simulink model "test_mdl_NI"  (R2018a)
settings: Solver=VariableStepAuto  StartTime=0.0  StopTime=10.0  RelTol=1e-3
(part 19 of 24)

== system test_mdl_NI/CAN_Signal/GWM/Other_GWMTx/Cluster_Info1_FD1 ==
  in : Inport
  AccDeny_B_RqIpc : Subsystem
  AccEnbl_B_RqDrv : Subsystem
  BulbChkActv_B_Stat : Subsystem
  DrvPerfMde_D_Rq : Subsystem
  DrvSlipCtlMde_B_Rq2 : Subsystem
  DrvSlipCtlMde_D_Rq : Subsystem
  EmgcyCallAsstMykey_Rq : Subsystem
  EngIdlShutDown_B_RqDrv : Subsystem
  EngOilLife_B_RqReset : Subsystem
  Fda_B_Stat : Subsystem
  FrostWarn_D_Stat : Subsystem
  HsaMde_D_Rq : Subsystem
  KeyTypeChngMykey_D_Rq : Subsystem
  LscmbbStat_B_Actl : Subsystem
  ManRgen_D_Rq : Subsystem
  MetricActvTe_B_Actl : Subsystem
  MetricActv_B_Actl : Subsystem
  NtrlTowMdeEnbl_B_RqDrv : Subsystem
  OdometerMasterValue : Subsystem
  ParkDetect_Stat : Subsystem
  Power_Liftgate_Mode_Cmd : Subsystem
  PrkLckCtlEnbl_D_RqIpc : Subsystem
  PtDrvMde_D_Rq : Subsystem
  ReducedGuard_D_Rq : Subsystem
  StopStrtDrvMde_D_RqMnu : Subsystem
  TRAILER_BRAKE_CONFIG : Subsystem
  TRLR_SWAY_CONFIG_CMD : Subsystem
  TrlrBrkMde_D_Rq : Subsystem
  bus_creator : BusCreator  Inputs=29
  bus_selector : BusSelector  OutputSignals=AccDeny_B_RqIpc,AccEnbl_B_RqDrv,BulbChkActv_B_Stat,DrvPerfMde_D_Rq,DrvSlipCtlMde_B_Rq2,DrvSlipCtlMde_D_Rq,EmgcyCallAsstMykey_Rq,EngIdlShutDown_B_RqDrv,EngOilLife_B_RqReset,Fda_B_Stat,FrostWarn_D_Stat,HsaMde_D_Rq,KeyTypeChngMykey_D_Rq,LscmbbStat_B_Actl,ManRgen_D_Rq,MetricActvTe_B_Actl,MetricActv_B_Actl,NtrlTowMdeEnbl_B_RqDrv,OdometerMasterValue,ParkDetect_Stat,Power_Liftgate_Mode_Cmd,PrkLckCtlEnbl_D_RqIpc,PtDrvMde_D_Rq,ReducedGuard_D_Rq,StopStrtDrvMde_D_RqMnu,TRAILER_BRAKE_CONFIG,TRLR_SWAY_CONFIG_CMD,TrlrBrkMde_D_Rq,ePRNDL_MODE
  ePRNDL_MODE : Subsystem
  out_port : Outport
  wires:
  bus_creator/1 -> out_port/1  "Cluster_Info1_FD1"
  AccDeny_B_RqIpc/1(out) -> bus_creator/1  "AccDeny_B_RqIpc"
  AccEnbl_B_RqDrv/1(out) -> bus_creator/2  "AccEnbl_B_RqDrv"
  BulbChkActv_B_Stat/1(out) -> bus_creator/3  "BulbChkActv_B_Stat"
  DrvPerfMde_D_Rq/1(out) -> bus_creator/4  "DrvPerfMde_D_Rq"
  DrvSlipCtlMde_B_Rq2/1(out) -> bus_creator/5  "DrvSlipCtlMde_B_Rq2"
  DrvSlipCtlMde_D_Rq/1(out) -> bus_creator/6  "DrvSlipCtlMde_D_Rq"
  EmgcyCallAsstMykey_Rq/1(out) -> bus_creator/7  "EmgcyCallAsstMykey_Rq"
  EngIdlShutDown_B_RqDrv/1(out) -> bus_creator/8  "EngIdlShutDown_B_RqDrv"
  EngOilLife_B_RqReset/1(out) -> bus_creator/9  "EngOilLife_B_RqReset"
  Fda_B_Stat/1(out) -> bus_creator/10  "Fda_B_Stat"
  FrostWarn_D_Stat/1(out) -> bus_creator/11  "FrostWarn_D_Stat"
  HsaMde_D_Rq/1(out) -> bus_creator/12  "HsaMde_D_Rq"
  KeyTypeChngMykey_D_Rq/1(out) -> bus_creator/13  "KeyTypeChngMykey_D_Rq"
  LscmbbStat_B_Actl/1(out) -> bus_creator/14  "LscmbbStat_B_Actl"
  ManRgen_D_Rq/1(out) -> bus_creator/15  "ManRgen_D_Rq"
  MetricActvTe_B_Actl/1(out) -> bus_creator/16  "MetricActvTe_B_Actl"
  MetricActv_B_Actl/1(out) -> bus_creator/17  "MetricActv_B_Actl"
  NtrlTowMdeEnbl_B_RqDrv/1(out) -> bus_creator/18  "NtrlTowMdeEnbl_B_RqDrv"
  OdometerMasterValue/1(out) -> bus_creator/19  "OdometerMasterValue"
  ParkDetect_Stat/1(out) -> bus_creator/20  "ParkDetect_Stat"
  Power_Liftgate_Mode_Cmd/1(out) -> bus_creator/21  "Power_Liftgate_Mode_Cmd"
  PrkLckCtlEnbl_D_RqIpc/1(out) -> bus_creator/22  "PrkLckCtlEnbl_D_RqIpc"
  PtDrvMde_D_Rq/1(out) -> bus_creator/23  "PtDrvMde_D_Rq"
  ReducedGuard_D_Rq/1(out) -> bus_creator/24  "ReducedGuard_D_Rq"
  StopStrtDrvMde_D_RqMnu/1(out) -> bus_creator/25  "StopStrtDrvMde_D_RqMnu"
  TRAILER_BRAKE_CONFIG/1(out) -> bus_creator/26  "TRAILER_BRAKE_CONFIG"
  TRLR_SWAY_CONFIG_CMD/1(out) -> bus_creator/27  "TRLR_SWAY_CONFIG_CMD"
  TrlrBrkMde_D_Rq/1(out) -> bus_creator/28  "TrlrBrkMde_D_Rq"
  ePRNDL_MODE/1(out) -> bus_creator/29  "ePRNDL_MODE"
  bus_selector/1 -> AccDeny_B_RqIpc/1(in)  "<AccDeny_B_RqIpc>"
  bus_selector/2 -> AccEnbl_B_RqDrv/1(in)  "<AccEnbl_B_RqDrv>"
  bus_selector/3 -> BulbChkActv_B_Stat/1(in)  "<BulbChkActv_B_Stat>"
  bus_selector/4 -> DrvPerfMde_D_Rq/1(in)  "<DrvPerfMde_D_Rq>"
  bus_selector/5 -> DrvSlipCtlMde_B_Rq2/1(in)  "<DrvSlipCtlMde_B_Rq2>"
  bus_selector/6 -> DrvSlipCtlMde_D_Rq/1(in)  "<DrvSlipCtlMde_D_Rq>"
  bus_selector/7 -> EmgcyCallAsstMykey_Rq/1(in)  "<EmgcyCallAsstMykey_Rq>"
  bus_selector/8 -> EngIdlShutDown_B_RqDrv/1(in)  "<EngIdlShutDown_B_RqDrv>"
  bus_selector/9 -> EngOilLife_B_RqReset/1(in)  "<EngOilLife_B_RqReset>"
  bus_selector/10 -> Fda_B_Stat/1(in)  "<Fda_B_Stat>"
  bus_selector/11 -> FrostWarn_D_Stat/1(in)  "<FrostWarn_D_Stat>"
  bus_selector/12 -> HsaMde_D_Rq/1(in)  "<HsaMde_D_Rq>"
  bus_selector/13 -> KeyTypeChngMykey_D_Rq/1(in)  "<KeyTypeChngMykey_D_Rq>"
  bus_selector/14 -> LscmbbStat_B_Actl/1(in)  "<LscmbbStat_B_Actl>"
  bus_selector/15 -> ManRgen_D_Rq/1(in)  "<ManRgen_D_Rq>"
  bus_selector/16 -> MetricActvTe_B_Actl/1(in)  "<MetricActvTe_B_Actl>"
  bus_selector/17 -> MetricActv_B_Actl/1(in)  "<MetricActv_B_Actl>"
  bus_selector/18 -> NtrlTowMdeEnbl_B_RqDrv/1(in)  "<NtrlTowMdeEnbl_B_RqDrv>"
  bus_selector/19 -> OdometerMasterValue/1(in)  "<OdometerMasterValue>"
  bus_selector/20 -> ParkDetect_Stat/1(in)  "<ParkDetect_Stat>"
  bus_selector/21 -> Power_Liftgate_Mode_Cmd/1(in)  "<Power_Liftgate_Mode_Cmd>"
  bus_selector/22 -> PrkLckCtlEnbl_D_RqIpc/1(in)  "<PrkLckCtlEnbl_D_RqIpc>"
  bus_selector/23 -> PtDrvMde_D_Rq/1(in)  "<PtDrvMde_D_Rq>"
  bus_selector/24 -> ReducedGuard_D_Rq/1(in)  "<ReducedGuard_D_Rq>"
  bus_selector/25 -> StopStrtDrvMde_D_RqMnu/1(in)  "<StopStrtDrvMde_D_RqMnu>"
  bus_selector/26 -> TRAILER_BRAKE_CONFIG/1(in)  "<TRAILER_BRAKE_CONFIG>"
  bus_selector/27 -> TRLR_SWAY_CONFIG_CMD/1(in)  "<TRLR_SWAY_CONFIG_CMD>"
  bus_selector/28 -> TrlrBrkMde_D_Rq/1(in)  "<TrlrBrkMde_D_Rq>"
  bus_selector/29 -> ePRNDL_MODE/1(in)  "<ePRNDL_MODE>"
  in/1 -> bus_selector/1

== system test_mdl_NI/CAN_Signal/GWM/Other_GWMTx/Cluster_Info_3_FD1 ==
  in : Inport
  AutoRgen_D_Rq : Subsystem
  DISPLAY_SPEED_OFFSET : Subsystem
  DISPLAY_SPEED_SCALING : Subsystem
  DrvSlipCtlMde_B_RqMyKey : Subsystem
  FUEL_SENSOR_NUM : Subsystem
  FuelLvlActvSide_No_Raw : Subsystem
  FuelLvlPssvSide_No_Raw : Subsystem
  FuelLvlWarn_D_Actl : Subsystem
  FuelLvl_Pc_Dsply : Subsystem
  FuelSecndActv_B_Actl : Subsystem
  OdoTripRx_B_Actl : Subsystem
  Veh_V_CompLimMx : Subsystem
  W2S_LAMP_OK : Subsystem
  bus_creator : BusCreator  Inputs=13
  bus_selector : BusSelector  OutputSignals=AutoRgen_D_Rq,DISPLAY_SPEED_OFFSET,DISPLAY_SPEED_SCALING,DrvSlipCtlMde_B_RqMyKey,FUEL_SENSOR_NUM,FuelLvlActvSide_No_Raw,FuelLvlPssvSide_No_Raw,FuelLvlWarn_D_Actl,FuelLvl_Pc_Dsply,FuelSecndActv_B_Actl,OdoTripRx_B_Actl,Veh_V_CompLimMx,W2S_LAMP_OK
  out_port : Outport
  wires:
  bus_creator/1 -> out_port/1  "Cluster_Info_3_FD1"
  AutoRgen_D_Rq/1(out) -> bus_creator/1  "AutoRgen_D_Rq"
  DISPLAY_SPEED_OFFSET/1(out) -> bus_creator/2  "DISPLAY_SPEED_OFFSET"
  DISPLAY_SPEED_SCALING/1(out) -> bus_creator/3  "DISPLAY_SPEED_SCALING"
  DrvSlipCtlMde_B_RqMyKey/1(out) -> bus_creator/4  "DrvSlipCtlMde_B_RqMyKey"
  FUEL_SENSOR_NUM/1(out) -> bus_creator/5  "FUEL_SENSOR_NUM"
  FuelLvlActvSide_No_Raw/1(out) -> bus_creator/6  "FuelLvlActvSide_No_Raw"
  FuelLvlPssvSide_No_Raw/1(out) -> bus_creator/7  "FuelLvlPssvSide_No_Raw"
  FuelLvlWarn_D_Actl/1(out) -> bus_creator/8  "FuelLvlWarn_D_Actl"
  FuelLvl_Pc_Dsply/1(out) -> bus_creator/9  "FuelLvl_Pc_Dsply"
  FuelSecndActv_B_Actl/1(out) -> bus_creator/10  "FuelSecndActv_B_Actl"
  OdoTripRx_B_Actl/1(out) -> bus_creator/11  "OdoTripRx_B_Actl"
  Veh_V_CompLimMx/1(out) -> bus_creator/12  "Veh_V_CompLimMx"
  W2S_LAMP_OK/1(out) -> bus_creator/13  "W2S_LAMP_OK"
  bus_selector/1 -> AutoRgen_D_Rq/1(in)  "<AutoRgen_D_Rq>"
  bus_selector/2 -> DISPLAY_SPEED_OFFSET/1(in)  "<DISPLAY_SPEED_OFFSET>"
  bus_selector/3 -> DISPLAY_SPEED_SCALING/1(in)  "<DISPLAY_SPEED_SCALING>"
  bus_selector/4 -> DrvSlipCtlMde_B_RqMyKey/1(in)  "<DrvSlipCtlMde_B_RqMyKey>"
  bus_selector/5 -> FUEL_SENSOR_NUM/1(in)  "<FUEL_SENSOR_NUM>"
  bus_selector/6 -> FuelLvlActvSide_No_Raw/1(in)  "<FuelLvlActvSide_No_Raw>"
  bus_selector/7 -> FuelLvlPssvSide_No_Raw/1(in)  "<FuelLvlPssvSide_No_Raw>"
  bus_selector/8 -> FuelLvlWarn_D_Actl/1(in)  "<FuelLvlWarn_D_Actl>"
  bus_selector/9 -> FuelLvl_Pc_Dsply/1(in)  "<FuelLvl_Pc_Dsply>"
  bus_selector/10 -> FuelSecndActv_B_Actl/1(in)  "<FuelSecndActv_B_Actl>"
  bus_selector/11 -> OdoTripRx_B_Actl/1(in)  "<OdoTripRx_B_Actl>"
  bus_selector/12 -> Veh_V_CompLimMx/1(in)  "<Veh_V_CompLimMx>"
  bus_selector/13 -> W2S_LAMP_OK/1(in)  "<W2S_LAMP_OK>"
  in/1 -> bus_selector/1

== system test_mdl_NI/CAN_Signal/GWM/Other_GWMTx/Cluster_Lighting_Rq_FD1 ==
  in : Inport
  IsaOffst_D_Rq : Subsystem
  SlMde_D_Rq : Subsystem
  bus_creator : BusCreator  Inputs=2
  bus_selector : BusSelector  OutputSignals=IsaOffst_D_Rq,SlMde_D_Rq
  out_port : Outport
  wires:
  bus_creator/1 -> out_port/1  "Cluster_Lighting_Rq_FD1"
  IsaOffst_D_Rq/1(out) -> bus_creator/1  "IsaOffst_D_Rq"
  SlMde_D_Rq/1(out) -> bus_creator/2  "SlMde_D_Rq"
  bus_selector/1 -> IsaOffst_D_Rq/1(in)  "<IsaOffst_D_Rq>"
  bus_selector/2 -> SlMde_D_Rq/1(in)  "<SlMde_D_Rq>"
  in/1 -> bus_selector/1

== system test_mdl_NI/CAN_Signal/GWM/Other_GWMTx/Compressor_Req_FD1 ==
  in : Inport
  ClimtCoolRear_B_Rq : Subsystem
  ClimtCool_D_Rq : Subsystem
  ClimtDeltaLoad_Pw_Actl : Subsystem
  ClimtHeatRear_D_Rq : Subsystem
  ClimtHeat_D_Rq : Subsystem
  ClimtPw_B_Rq : Subsystem
  HtrCorePump_B_Rq : Subsystem
  HvacAirCond_B_Rq : Subsystem
  HvacEvap_Te_Actl : Subsystem
  HvacEvap_Te_Offst : Subsystem
  HvacEvap_Te_Rq : Subsystem
  HvacHtrCore_Te_Rq : Subsystem
  SnowPlowMde_B_Enbl : Subsystem
  StopStrtDrvMde_B_RqBtn : Subsystem
  WndwFrontHeat_B_Stat : Subsystem
  bus_creator : BusCreator  Inputs=15
  bus_selector : BusSelector  OutputSignals=ClimtCoolRear_B_Rq,ClimtCool_D_Rq,ClimtDeltaLoad_Pw_Actl,ClimtHeatRear_D_Rq,ClimtHeat_D_Rq,ClimtPw_B_Rq,HtrCorePump_B_Rq,HvacAirCond_B_Rq,HvacEvap_Te_Actl,HvacEvap_Te_Offst,HvacEvap_Te_Rq,HvacHtrCore_Te_Rq,SnowPlowMde_B_Enbl,StopStrtDrvMde_B_RqBtn,WndwFrontHeat_B_Stat
  out_port : Outport
  wires:
  bus_creator/1 -> out_port/1  "Compressor_Req_FD1"
  ClimtCoolRear_B_Rq/1(out) -> bus_creator/1  "ClimtCoolRear_B_Rq"
  ClimtCool_D_Rq/1(out) -> bus_creator/2  "ClimtCool_D_Rq"
  ClimtDeltaLoad_Pw_Actl/1(out) -> bus_creator/3  "ClimtDeltaLoad_Pw_Actl"
  ClimtHeatRear_D_Rq/1(out) -> bus_creator/4  "ClimtHeatRear_D_Rq"
  ClimtHeat_D_Rq/1(out) -> bus_creator/5  "ClimtHeat_D_Rq"
  ClimtPw_B_Rq/1(out) -> bus_creator/6  "ClimtPw_B_Rq"
  HtrCorePump_B_Rq/1(out) -> bus_creator/7  "HtrCorePump_B_Rq"
  HvacAirCond_B_Rq/1(out) -> bus_creator/8  "HvacAirCond_B_Rq"
  HvacEvap_Te_Actl/1(out) -> bus_creator/9  "HvacEvap_Te_Actl"
  HvacEvap_Te_Offst/1(out) -> bus_creator/10  "HvacEvap_Te_Offst"
  HvacEvap_Te_Rq/1(out) -> bus_creator/11  "HvacEvap_Te_Rq"
  HvacHtrCore_Te_Rq/1(out) -> bus_creator/12  "HvacHtrCore_Te_Rq"
  SnowPlowMde_B_Enbl/1(out) -> bus_creator/13  "SnowPlowMde_B_Enbl"
  StopStrtDrvMde_B_RqBtn/1(out) -> bus_creator/14  "StopStrtDrvMde_B_RqBtn"
  WndwFrontHeat_B_Stat/1(out) -> bus_creator/15  "WndwFrontHeat_B_Stat"
  bus_selector/1 -> ClimtCoolRear_B_Rq/1(in)  "<ClimtCoolRear_B_Rq>"
  bus_selector/2 -> ClimtCool_D_Rq/1(in)  "<ClimtCool_D_Rq>"
  bus_selector/3 -> ClimtDeltaLoad_Pw_Actl/1(in)  "<ClimtDeltaLoad_Pw_Actl>"
  bus_selector/4 -> ClimtHeatRear_D_Rq/1(in)  "<ClimtHeatRear_D_Rq>"
  bus_selector/5 -> ClimtHeat_D_Rq/1(in)  "<ClimtHeat_D_Rq>"
  bus_selector/6 -> ClimtPw_B_Rq/1(in)  "<ClimtPw_B_Rq>"
  bus_selector/7 -> HtrCorePump_B_Rq/1(in)  "<HtrCorePump_B_Rq>"
  bus_selector/8 -> HvacAirCond_B_Rq/1(in)  "<HvacAirCond_B_Rq>"
  bus_selector/9 -> HvacEvap_Te_Actl/1(in)  "<HvacEvap_Te_Actl>"
  bus_selector/10 -> HvacEvap_Te_Offst/1(in)  "<HvacEvap_Te_Offst>"
  bus_selector/11 -> HvacEvap_Te_Rq/1(in)  "<HvacEvap_Te_Rq>"
  bus_selector/12 -> HvacHtrCore_Te_Rq/1(in)  "<HvacHtrCore_Te_Rq>"
  bus_selector/13 -> SnowPlowMde_B_Enbl/1(in)  "<SnowPlowMde_B_Enbl>"
  bus_selector/14 -> StopStrtDrvMde_B_RqBtn/1(in)  "<StopStrtDrvMde_B_RqBtn>"
  bus_selector/15 -> WndwFrontHeat_B_Stat/1(in)  "<WndwFrontHeat_B_Stat>"
  in/1 -> bus_selector/1

== system test_mdl_NI/CAN_Signal/GWM/Other_GWMTx/CruiseCtrl_Strg_Data_FD1 ==
  in : Inport
  AccButtnGapDecPress2 : Subsystem
  AccButtnGapIncPress2 : Subsystem
  AccButtnGpTogglePress2 : Subsystem
  ActvFrontSteLck_D_Stat : Subsystem
  ActvFrontSteMsgTxt_D_Rq : Subsystem
  AslButtnOnOffCnclPres2 : Subsystem
  AslButtnOnOffPress2 : Subsystem
  CcAslButtnCnclPress2 : Subsystem
  CcAslButtnCnclResPres2 : Subsystem
  CcAslButtnDeny_B_Actl2 : Subsystem
  CcAslButtnIndxDecPres2 : Subsystem
  CcAslButtnIndxIncPres2 : Subsystem
  CcAslButtnOffCnclPres2 : Subsystem
  CcAslButtnOnOffCncl2 : Subsystem
  CcAslButtnOnPress2 : Subsystem
  CcAslButtnResDecPress2 : Subsystem
  CcAslButtnResIncPress2 : Subsystem
  CcAslButtnSetDecPress2 : Subsystem
  CcAslButtnSetIncPress2 : Subsystem
  CcAslButtnSetPress2 : Subsystem
  CcAsllButtnResPress2 : Subsystem
  CcButtnOffPress2 : Subsystem
  CcButtnOnOffCnclPress2 : Subsystem
  CcButtnOnOffPress2 : Subsystem
  CcButtnOnPress2 : Subsystem
  SelDrvMdeAdptSte_D_Stat : Subsystem
  TjaButtnOnOffPress2 : Subsystem
  bus_creator : BusCreator  Inputs=27
  bus_selector : BusSelector  OutputSignals=AccButtnGapDecPress2,AccButtnGapIncPress2,AccButtnGpTogglePress2,ActvFrontSteLck_D_Stat,ActvFrontSteMsgTxt_D_Rq,AslButtnOnOffCnclPres2,AslButtnOnOffPress2,CcAslButtnCnclPress2,CcAslButtnCnclResPres2,CcAslButtnDeny_B_Actl2,CcAslButtnIndxDecPres2,CcAslButtnIndxIncPres2,CcAslButtnOffCnclPres2,CcAslButtnOnOffCncl2,CcAslButtnOnPress2,CcAslButtnResDecPress2,CcAslButtnResIncPress2,CcAslButtnSetDecPress2,CcAslButtnSetIncPress2,CcAslButtnSetPress2,CcAsllButtnResPress2,CcButtnOffPress2,CcButtnOnOffCnclPress2,CcButtnOnOffPress2,CcButtnOnPress2,SelDrvMdeAdptSte_D_Stat,TjaButtnOnOffPress2
  out_port : Outport
  wires:
  bus_creator/1 -> out_port/1  "CruiseCtrl_Strg_Data_FD1"
  AccButtnGapDecPress2/1(out) -> bus_creator/1  "AccButtnGapDecPress2"
  AccButtnGapIncPress2/1(out) -> bus_creator/2  "AccButtnGapIncPress2"
  AccButtnGpTogglePress2/1(out) -> bus_creator/3  "AccButtnGpTogglePress2"
  ActvFrontSteLck_D_Stat/1(out) -> bus_creator/4  "ActvFrontSteLck_D_Stat"
  ActvFrontSteMsgTxt_D_Rq/1(out) -> bus_creator/5  "ActvFrontSteMsgTxt_D_Rq"
  AslButtnOnOffCnclPres2/1(out) -> bus_creator/6  "AslButtnOnOffCnclPres2"
  AslButtnOnOffPress2/1(out) -> bus_creator/7  "AslButtnOnOffPress2"
  CcAslButtnCnclPress2/1(out) -> bus_creator/8  "CcAslButtnCnclPress2"
  CcAslButtnCnclResPres2/1(out) -> bus_creator/9  "CcAslButtnCnclResPres2"
  CcAslButtnDeny_B_Actl2/1(out) -> bus_creator/10  "CcAslButtnDeny_B_Actl2"
  CcAslButtnIndxDecPres2/1(out) -> bus_creator/11  "CcAslButtnIndxDecPres2"
  CcAslButtnIndxIncPres2/1(out) -> bus_creator/12  "CcAslButtnIndxIncPres2"
  CcAslButtnOffCnclPres2/1(out) -> bus_creator/13  "CcAslButtnOffCnclPres2"
  CcAslButtnOnOffCncl2/1(out) -> bus_creator/14  "CcAslButtnOnOffCncl2"
  CcAslButtnOnPress2/1(out) -> bus_creator/15  "CcAslButtnOnPress2"
  CcAslButtnResDecPress2/1(out) -> bus_creator/16  "CcAslButtnResDecPress2"
  CcAslButtnResIncPress2/1(out) -> bus_creator/17  "CcAslButtnResIncPress2"
  CcAslButtnSetDecPress2/1(out) -> bus_creator/18  "CcAslButtnSetDecPress2"
  CcAslButtnSetIncPress2/1(out) -> bus_creator/19  "CcAslButtnSetIncPress2"
  CcAslButtnSetPress2/1(out) -> bus_creator/20  "CcAslButtnSetPress2"
  CcAsllButtnResPress2/1(out) -> bus_creator/21  "CcAsllButtnResPress2"
  CcButtnOffPress2/1(out) -> bus_creator/22  "CcButtnOffPress2"
  CcButtnOnOffCnclPress2/1(out) -> bus_creator/23  "CcButtnOnOffCnclPress2"
  CcButtnOnOffPress2/1(out) -> bus_creator/24  "CcButtnOnOffPress2"
  CcButtnOnPress2/1(out) -> bus_creator/25  "CcButtnOnPress2"
  SelDrvMdeAdptSte_D_Stat/1(out) -> bus_creator/26  "SelDrvMdeAdptSte_D_Stat"
  TjaButtnOnOffPress2/1(out) -> bus_creator/27  "TjaButtnOnOffPress2"
  bus_selector/1 -> AccButtnGapDecPress2/1(in)  "<AccButtnGapDecPress2>"
  bus_selector/2 -> AccButtnGapIncPress2/1(in)  "<AccButtnGapIncPress2>"
  bus_selector/3 -> AccButtnGpTogglePress2/1(in)  "<AccButtnGpTogglePress2>"
  bus_selector/4 -> ActvFrontSteLck_D_Stat/1(in)  "<ActvFrontSteLck_D_Stat>"
  bus_selector/5 -> ActvFrontSteMsgTxt_D_Rq/1(in)  "<ActvFrontSteMsgTxt_D_Rq>"
  bus_selector/6 -> AslButtnOnOffCnclPres2/1(in)  "<AslButtnOnOffCnclPres2>"
  bus_selector/7 -> AslButtnOnOffPress2/1(in)  "<AslButtnOnOffPress2>"
  bus_selector/8 -> CcAslButtnCnclPress2/1(in)  "<CcAslButtnCnclPress2>"
  bus_selector/9 -> CcAslButtnCnclResPres2/1(in)  "<CcAslButtnCnclResPres2>"
  bus_selector/10 -> CcAslButtnDeny_B_Actl2/1(in)  "<CcAslButtnDeny_B_Actl2>"
  bus_selector/11 -> CcAslButtnIndxDecPres2/1(in)  "<CcAslButtnIndxDecPres2>"
  bus_selector/12 -> CcAslButtnIndxIncPres2/1(in)  "<CcAslButtnIndxIncPres2>"
  bus_selector/13 -> CcAslButtnOffCnclPres2/1(in)  "<CcAslButtnOffCnclPres2>"
  bus_selector/14 -> CcAslButtnOnOffCncl2/1(in)  "<CcAslButtnOnOffCncl2>"
  bus_selector/15 -> CcAslButtnOnPress2/1(in)  "<CcAslButtnOnPress2>"
  bus_selector/16 -> CcAslButtnResDecPress2/1(in)  "<CcAslButtnResDecPress2>"
  bus_selector/17 -> CcAslButtnResIncPress2/1(in)  "<CcAslButtnResIncPress2>"
  bus_selector/18 -> CcAslButtnSetDecPress2/1(in)  "<CcAslButtnSetDecPress2>"
  bus_selector/19 -> CcAslButtnSetIncPress2/1(in)  "<CcAslButtnSetIncPress2>"
  bus_selector/20 -> CcAslButtnSetPress2/1(in)  "<CcAslButtnSetPress2>"
  bus_selector/21 -> CcAsllButtnResPress2/1(in)  "<CcAsllButtnResPress2>"
  bus_selector/22 -> CcButtnOffPress2/1(in)  "<CcButtnOffPress2>"
  bus_selector/23 -> CcButtnOnOffCnclPress2/1(in)  "<CcButtnOnOffCnclPress2>"
  bus_selector/24 -> CcButtnOnOffPress2/1(in)  "<CcButtnOnOffPress2>"
  bus_selector/25 -> CcButtnOnPress2/1(in)  "<CcButtnOnPress2>"
  bus_selector/26 -> SelDrvMdeAdptSte_D_Stat/1(in)  "<SelDrvMdeAdptSte_D_Stat>"
  bus_selector/27 -> TjaButtnOnOffPress2/1(in)  "<TjaButtnOnOffPress2>"
  in/1 -> bus_selector/1

== system test_mdl_NI/CAN_Signal/GWM/Other_GWMTx/DCACA_Data1_FD1 ==
  in : Inport
  CoolFanDcac_D_Rq : Subsystem
  DcacClntFlw_D_Rq : Subsystem
  DcacPlugPrsnt_B_Stat : Subsystem
  DcacRdy_D_Stat : Subsystem
  bus_creator : BusCreator  Inputs=4
  bus_selector : BusSelector  OutputSignals=CoolFanDcac_D_Rq,DcacClntFlw_D_Rq,DcacPlugPrsnt_B_Stat,DcacRdy_D_Stat
  out_port : Outport
  wires:
  bus_creator/1 -> out_port/1  "DCACA_Data1_FD1"
  CoolFanDcac_D_Rq/1(out) -> bus_creator/1  "CoolFanDcac_D_Rq"
  DcacClntFlw_D_Rq/1(out) -> bus_creator/2  "DcacClntFlw_D_Rq"
  DcacPlugPrsnt_B_Stat/1(out) -> bus_creator/3  "DcacPlugPrsnt_B_Stat"
  DcacRdy_D_Stat/1(out) -> bus_creator/4  "DcacRdy_D_Stat"
  bus_selector/1 -> CoolFanDcac_D_Rq/1(in)  "<CoolFanDcac_D_Rq>"
  bus_selector/2 -> DcacClntFlw_D_Rq/1(in)  "<DcacClntFlw_D_Rq>"
  bus_selector/3 -> DcacPlugPrsnt_B_Stat/1(in)  "<DcacPlugPrsnt_B_Stat>"
  bus_selector/4 -> DcacRdy_D_Stat/1(in)  "<DcacRdy_D_Stat>"
  in/1 -> bus_selector/1

== system test_mdl_NI/CAN_Signal/GWM/Other_GWMTx/DCACA_Data2_FD1 ==
  in : Inport
  DcacIn_I_Actl : Subsystem
  DcacIn_U_Actl : Subsystem
  Dcac_Te_Actl : Subsystem
  bus_creator : BusCreator  Inputs=3
  bus_selector : BusSelector  OutputSignals=DcacIn_I_Actl,DcacIn_U_Actl,Dcac_Te_Actl
  out_port : Outport
  wires:
  bus_creator/1 -> out_port/1  "DCACA_Data2_FD1"
  DcacIn_I_Actl/1(out) -> bus_creator/1  "DcacIn_I_Actl"
  DcacIn_U_Actl/1(out) -> bus_creator/2  "DcacIn_U_Actl"
  Dcac_Te_Actl/1(out) -> bus_creator/3  "Dcac_Te_Actl"
  bus_selector/1 -> DcacIn_I_Actl/1(in)  "<DcacIn_I_Actl>"
  bus_selector/2 -> DcacIn_U_Actl/1(in)  "<DcacIn_U_Actl>"
  bus_selector/3 -> Dcac_Te_Actl/1(in)  "<Dcac_Te_Actl>"
  in/1 -> bus_selector/1

== system test_mdl_NI/CAN_Signal/GWM/Other_GWMTx/DCACA_Data3_FD1 ==
  in : Inport
  DcacIn_Pw_Mx : Subsystem
  DcacOut1_Pw_Actl : Subsystem
  DcacOut2_Pw_Actl : Subsystem
  DcacOut_Pw_Mx : Subsystem
  bus_creator : BusCreator  Inputs=4
  bus_selector : BusSelector  OutputSignals=DcacIn_Pw_Mx,DcacOut1_Pw_Actl,DcacOut2_Pw_Actl,DcacOut_Pw_Mx
  out_port : Outport
  wires:
  bus_creator/1 -> out_port/1  "DCACA_Data3_FD1"
  DcacIn_Pw_Mx/1(out) -> bus_creator/1  "DcacIn_Pw_Mx"
  DcacOut1_Pw_Actl/1(out) -> bus_creator/2  "DcacOut1_Pw_Actl"
  DcacOut2_Pw_Actl/1(out) -> bus_creator/3  "DcacOut2_Pw_Actl"
  DcacOut_Pw_Mx/1(out) -> bus_creator/4  "DcacOut_Pw_Mx"
  bus_selector/1 -> DcacIn_Pw_Mx/1(in)  "<DcacIn_Pw_Mx>"
  bus_selector/2 -> DcacOut1_Pw_Actl/1(in)  "<DcacOut1_Pw_Actl>"
  bus_selector/3 -> DcacOut2_Pw_Actl/1(in)  "<DcacOut2_Pw_Actl>"
  bus_selector/4 -> DcacOut_Pw_Mx/1(in)  "<DcacOut_Pw_Mx>"
  in/1 -> bus_selector/1

== system test_mdl_NI/CAN_Signal/GWM/Other_GWMTx/DifferentialCtrlData_1_FD1 ==
  in : Inport
  RearDiffLck_Tq_Actl2 : Subsystem
  bus_creator : BusCreator  Inputs=1
  bus_selector : BusSelector  OutputSignals=RearDiffLck_Tq_Actl2
  out_port : Outport
  wires:
  bus_creator/1 -> out_port/1  "DifferentialCtrlData_1_FD1"
  RearDiffLck_Tq_Actl2/1(out) -> bus_creator/1  "RearDiffLck_Tq_Actl2"
  bus_selector/1 -> RearDiffLck_Tq_Actl2/1(in)  "<RearDiffLck_Tq_Actl2>"
  in/1 -> bus_selector/1

== system test_mdl_NI/CAN_Signal/GWM/Other_GWMTx/Driver_Dr_Stat_FD1 ==
  in : Inport
  BLISLEDStatDriverSide : Subsystem
  ChildLckFdbckRd_B_Stat : Subsystem
  ChildLckPw_D_Rq : Subsystem
  ChildLckPw_N_Cnt : Subsystem
  Driver_Lock_Sw_Cnt : Subsystem
  Driver_Lock_Sw_Stat : Subsystem
  KeyCylSwDrvDr_D_Stat : Subsystem
  RollCodeDrvDrKeyCyl : Subsystem
  RvrseMirrorChime_B_Rq : Subsystem
  WndwDrvSide_D_Stat : Subsystem
  bus_creator : BusCreator  Inputs=10
  bus_selector : BusSelector  OutputSignals=BLISLEDStatDriverSide,ChildLckFdbckRd_B_Stat,ChildLckPw_D_Rq,ChildLckPw_N_Cnt,Driver_Lock_Sw_Cnt,Driver_Lock_Sw_Stat,KeyCylSwDrvDr_D_Stat,RollCodeDrvDrKeyCyl,RvrseMirrorChime_B_Rq,WndwDrvSide_D_Stat
  out_port : Outport
  wires:
  bus_creator/1 -> out_port/1  "Driver_Dr_Stat_FD1"
  BLISLEDStatDriverSide/1(out) -> bus_creator/1  "BLISLEDStatDriverSide"
  ChildLckFdbckRd_B_Stat/1(out) -> bus_creator/2  "ChildLckFdbckRd_B_Stat"
  ChildLckPw_D_Rq/1(out) -> bus_creator/3  "ChildLckPw_D_Rq"
  ChildLckPw_N_Cnt/1(out) -> bus_creator/4  "ChildLckPw_N_Cnt"
  Driver_Lock_Sw_Cnt/1(out) -> bus_creator/5  "Driver_Lock_Sw_Cnt"
  Driver_Lock_Sw_Stat/1(out) -> bus_creator/6  "Driver_Lock_Sw_Stat"
  KeyCylSwDrvDr_D_Stat/1(out) -> bus_creator/7  "KeyCylSwDrvDr_D_Stat"
  RollCodeDrvDrKeyCyl/1(out) -> bus_creator/8  "RollCodeDrvDrKeyCyl"
  RvrseMirrorChime_B_Rq/1(out) -> bus_creator/9  "RvrseMirrorChime_B_Rq"
  WndwDrvSide_D_Stat/1(out) -> bus_creator/10  "WndwDrvSide_D_Stat"
  bus_selector/1 -> BLISLEDStatDriverSide/1(in)  "<BLISLEDStatDriverSide>"
  bus_selector/2 -> ChildLckFdbckRd_B_Stat/1(in)  "<ChildLckFdbckRd_B_Stat>"
  bus_selector/3 -> ChildLckPw_D_Rq/1(in)  "<ChildLckPw_D_Rq>"
  bus_selector/4 -> ChildLckPw_N_Cnt/1(in)  "<ChildLckPw_N_Cnt>"
  bus_selector/5 -> Driver_Lock_Sw_Cnt/1(in)  "<Driver_Lock_Sw_Cnt>"
  bus_selector/6 -> Driver_Lock_Sw_Stat/1(in)  "<Driver_Lock_Sw_Stat>"
  bus_selector/7 -> KeyCylSwDrvDr_D_Stat/1(in)  "<KeyCylSwDrvDr_D_Stat>"
  bus_selector/8 -> RollCodeDrvDrKeyCyl/1(in)  "<RollCodeDrvDrKeyCyl>"
  bus_selector/9 -> RvrseMirrorChime_B_Rq/1(in)  "<RvrseMirrorChime_B_Rq>"
  bus_selector/10 -> WndwDrvSide_D_Stat/1(in)  "<WndwDrvSide_D_Stat>"
  in/1 -> bus_selector/1

== system test_mdl_NI/CAN_Signal/GWM/Other_GWMTx/Dsp_Request_Signals11_FD1 ==
  in : Inport
  ApaMdeStat_D_RqDrv : Subsystem
  ApaSwtch_D_RqMnu : Subsystem
  CamAutoTowbarZoom : Subsystem
  CamraOvrlDyn_D_Rq : Subsystem
  CamraOvrlStat_D_Rq : Subsystem
  CamraViewSplit_B_Rq : Subsystem
  CamraZoomMan_D_Rq : Subsystem
  DistanceBarSetting : Subsystem
  PrkAidSwtch_D_RqMnu : Subsystem
  bus_creator : BusCreator  Inputs=9
  bus_selector : BusSelector  OutputSignals=ApaMdeStat_D_RqDrv,ApaSwtch_D_RqMnu,CamAutoTowbarZoom,CamraOvrlDyn_D_Rq,CamraOvrlStat_D_Rq,CamraViewSplit_B_Rq,CamraZoomMan_D_Rq,DistanceBarSetting,PrkAidSwtch_D_RqMnu
  out_port : Outport
  wires:
  bus_creator/1 -> out_port/1  "Dsp_Request_Signals11_FD1"
  ApaMdeStat_D_RqDrv/1(out) -> bus_creator/1  "ApaMdeStat_D_RqDrv"
  ApaSwtch_D_RqMnu/1(out) -> bus_creator/2  "ApaSwtch_D_RqMnu"
  CamAutoTowbarZoom/1(out) -> bus_creator/3  "CamAutoTowbarZoom"
  CamraOvrlDyn_D_Rq/1(out) -> bus_creator/4  "CamraOvrlDyn_D_Rq"
  CamraOvrlStat_D_Rq/1(out) -> bus_creator/5  "CamraOvrlStat_D_Rq"
  CamraViewSplit_B_Rq/1(out) -> bus_creator/6  "CamraViewSplit_B_Rq"
  CamraZoomMan_D_Rq/1(out) -> bus_creator/7  "CamraZoomMan_D_Rq"
  DistanceBarSetting/1(out) -> bus_creator/8  "DistanceBarSetting"
  PrkAidSwtch_D_RqMnu/1(out) -> bus_creator/9  "PrkAidSwtch_D_RqMnu"
  bus_selector/1 -> ApaMdeStat_D_RqDrv/1(in)  "<ApaMdeStat_D_RqDrv>"
  bus_selector/2 -> ApaSwtch_D_RqMnu/1(in)  "<ApaSwtch_D_RqMnu>"
  bus_selector/3 -> CamAutoTowbarZoom/1(in)  "<CamAutoTowbarZoom>"
  bus_selector/4 -> CamraOvrlDyn_D_Rq/1(in)  "<CamraOvrlDyn_D_Rq>"
  bus_selector/5 -> CamraOvrlStat_D_Rq/1(in)  "<CamraOvrlStat_D_Rq>"
  bus_selector/6 -> CamraViewSplit_B_Rq/1(in)  "<CamraViewSplit_B_Rq>"
  bus_selector/7 -> CamraZoomMan_D_Rq/1(in)  "<CamraZoomMan_D_Rq>"
  bus_selector/8 -> DistanceBarSetting/1(in)  "<DistanceBarSetting>"
  bus_selector/9 -> PrkAidSwtch_D_RqMnu/1(in)  "<PrkAidSwtch_D_RqMnu>"
  in/1 -> bus_selector/1

== system test_mdl_NI/CAN_Signal/GWM/Other_GWMTx/ElecHorizon_Data1_FD1 ==
  in : Inport
  EhData1_No_Actl : Subsystem
  bus_creator : BusCreator  Inputs=1
  bus_selector : BusSelector  OutputSignals=EhData1_No_Actl
  out_port : Outport
  wires:
  bus_creator/1 -> out_port/1  "ElecHorizon_Data1_FD1"
  EhData1_No_Actl/1(out) -> bus_creator/1  "EhData1_No_Actl"
  bus_selector/1 -> EhData1_No_Actl/1(in)  "<EhData1_No_Actl>"
  in/1 -> bus_selector/1

== system test_mdl_NI/CAN_Signal/GWM/Other_GWMTx/ElecHorizon_Data2_FD1 ==
  in : Inport
  EhData2_No_Actl : Subsystem
  bus_creator : BusCreator  Inputs=1
  bus_selector : BusSelector  OutputSignals=EhData2_No_Actl
  out_port : Outport
  wires:
  bus_creator/1 -> out_port/1  "ElecHorizon_Data2_FD1"
  EhData2_No_Actl/1(out) -> bus_creator/1  "EhData2_No_Actl"
  bus_selector/1 -> EhData2_No_Actl/1(in)  "<EhData2_No_Actl>"
  in/1 -> bus_selector/1

== system test_mdl_NI/CAN_Signal/GWM/Other_GWMTx/FourByFourSwitchData_FD1 ==
  in : Inport
  AwdLck_D_RqDrv : Subsystem
  AwdMde_D_RqDrv : Subsystem
  DrvSlipCtlMde_B_Rq3 : Subsystem
  HdcSwtchPos_B_Actl : Subsystem
  HybMdeSwtch_B_Rq : Subsystem
  RearDiffLck_D_RqDrv : Subsystem
  TrailCtlSwtch_B_Stat3 : Subsystem
  bus_creator : BusCreator  Inputs=7
  bus_selector : BusSelector  OutputSignals=AwdLck_D_RqDrv,AwdMde_D_RqDrv,DrvSlipCtlMde_B_Rq3,HdcSwtchPos_B_Actl,HybMdeSwtch_B_Rq,RearDiffLck_D_RqDrv,TrailCtlSwtch_B_Stat3
  out_port : Outport
  wires:
  bus_creator/1 -> out_port/1  "FourByFourSwitchData_FD1"
  AwdLck_D_RqDrv/1(out) -> bus_creator/1  "AwdLck_D_RqDrv"
  AwdMde_D_RqDrv/1(out) -> bus_creator/2  "AwdMde_D_RqDrv"
  DrvSlipCtlMde_B_Rq3/1(out) -> bus_creator/3  "DrvSlipCtlMde_B_Rq3"
  HdcSwtchPos_B_Actl/1(out) -> bus_creator/4  "HdcSwtchPos_B_Actl"
  HybMdeSwtch_B_Rq/1(out) -> bus_creator/5  "HybMdeSwtch_B_Rq"
  RearDiffLck_D_RqDrv/1(out) -> bus_creator/6  "RearDiffLck_D_RqDrv"
  TrailCtlSwtch_B_Stat3/1(out) -> bus_creator/7  "TrailCtlSwtch_B_Stat3"
  bus_selector/1 -> AwdLck_D_RqDrv/1(in)  "<AwdLck_D_RqDrv>"
  bus_selector/2 -> AwdMde_D_RqDrv/1(in)  "<AwdMde_D_RqDrv>"
  bus_selector/3 -> DrvSlipCtlMde_B_Rq3/1(in)  "<DrvSlipCtlMde_B_Rq3>"
  bus_selector/4 -> HdcSwtchPos_B_Actl/1(in)  "<HdcSwtchPos_B_Actl>"
  bus_selector/5 -> HybMdeSwtch_B_Rq/1(in)  "<HybMdeSwtch_B_Rq>"
  bus_selector/6 -> RearDiffLck_D_RqDrv/1(in)  "<RearDiffLck_D_RqDrv>"
  bus_selector/7 -> TrailCtlSwtch_B_Stat3/1(in)  "<TrailCtlSwtch_B_Stat3>"
  in/1 -> bus_selector/1

== system test_mdl_NI/CAN_Signal/GWM/Other_GWMTx/Front_Distance_Req_FD1 ==
  in : Inport
  FdsmTrgCntr_B_Actl : Subsystem
  FdsmTrgDist_L_Actl : Subsystem
  FdsmTrgLeft_B_Actl : Subsystem
  FdsmTrgRight_B_Actl : Subsystem
  LscmbbBaSens_D_Rq : Subsystem
  LscmbbBlck_B_Actl : Subsystem
  LscmbbBrkDecel_A_Rq : Subsystem
  LscmbbBrkDecel_B_Enbl : Subsystem
  LscmbbBrkDecel_No_Cnt : Subsystem
  LscmbbBrkDecel_No_Cs : Subsystem
  LscmbbBrkPrchg_D_Rq : Subsystem
  LscmbbDeny_B_Actl : Subsystem
  LscmbbEngTqMn_B_Rq : Subsystem
  LscmbbMsgTxt_D_Rq : Subsystem
  LscmbbPostEvnt_B_Dsply : Subsystem
  LscmbbSrvcRqd_B_Rq : Subsystem
  WndwFrontHeat_B_Rq : Subsystem
  bus_creator : BusCreator  Inputs=17
  bus_selector : BusSelector  OutputSignals=FdsmTrgCntr_B_Actl,FdsmTrgDist_L_Actl,FdsmTrgLeft_B_Actl,FdsmTrgRight_B_Actl,LscmbbBaSens_D_Rq,LscmbbBlck_B_Actl,LscmbbBrkDecel_A_Rq,LscmbbBrkDecel_B_Enbl,LscmbbBrkDecel_No_Cnt,LscmbbBrkDecel_No_Cs,LscmbbBrkPrchg_D_Rq,LscmbbDeny_B_Actl,LscmbbEngTqMn_B_Rq,LscmbbMsgTxt_D_Rq,LscmbbPostEvnt_B_Dsply,LscmbbSrvcRqd_B_Rq,WndwFrontHeat_B_Rq
  out_port : Outport
  wires:
  bus_creator/1 -> out_port/1  "Front_Distance_Req_FD1"
  FdsmTrgCntr_B_Actl/1(out) -> bus_creator/1  "FdsmTrgCntr_B_Actl"
  FdsmTrgDist_L_Actl/1(out) -> bus_creator/2  "FdsmTrgDist_L_Actl"
  FdsmTrgLeft_B_Actl/1(out) -> bus_creator/3  "FdsmTrgLeft_B_Actl"
  FdsmTrgRight_B_Actl/1(out) -> bus_creator/4  "FdsmTrgRight_B_Actl"
  LscmbbBaSens_D_Rq/1(out) -> bus_creator/5  "LscmbbBaSens_D_Rq"
  LscmbbBlck_B_Actl/1(out) -> bus_creator/6  "LscmbbBlck_B_Actl"
  LscmbbBrkDecel_A_Rq/1(out) -> bus_creator/7  "LscmbbBrkDecel_A_Rq"
  LscmbbBrkDecel_B_Enbl/1(out) -> bus_creator/8  "LscmbbBrkDecel_B_Enbl"
  LscmbbBrkDecel_No_Cnt/1(out) -> bus_creator/9  "LscmbbBrkDecel_No_Cnt"
  LscmbbBrkDecel_No_Cs/1(out) -> bus_creator/10  "LscmbbBrkDecel_No_Cs"
  LscmbbBrkPrchg_D_Rq/1(out) -> bus_creator/11  "LscmbbBrkPrchg_D_Rq"
  LscmbbDeny_B_Actl/1(out) -> bus_creator/12  "LscmbbDeny_B_Actl"
  LscmbbEngTqMn_B_Rq/1(out) -> bus_creator/13  "LscmbbEngTqMn_B_Rq"
  LscmbbMsgTxt_D_Rq/1(out) -> bus_creator/14  "LscmbbMsgTxt_D_Rq"
  LscmbbPostEvnt_B_Dsply/1(out) -> bus_creator/15  "LscmbbPostEvnt_B_Dsply"
  LscmbbSrvcRqd_B_Rq/1(out) -> bus_creator/16  "LscmbbSrvcRqd_B_Rq"
  WndwFrontHeat_B_Rq/1(out) -> bus_creator/17  "WndwFrontHeat_B_Rq"
  bus_selector/1 -> FdsmTrgCntr_B_Actl/1(in)  "<FdsmTrgCntr_B_Actl>"
  bus_selector/2 -> FdsmTrgDist_L_Actl/1(in)  "<FdsmTrgDist_L_Actl>"
  bus_selector/3 -> FdsmTrgLeft_B_Actl/1(in)  "<FdsmTrgLeft_B_Actl>"
  bus_selector/4 -> FdsmTrgRight_B_Actl/1(in)  "<FdsmTrgRight_B_Actl>"
  bus_selector/5 -> LscmbbBaSens_D_Rq/1(in)  "<LscmbbBaSens_D_Rq>"
  bus_selector/6 -> LscmbbBlck_B_Actl/1(in)  "<LscmbbBlck_B_Actl>"
  bus_selector/7 -> LscmbbBrkDecel_A_Rq/1(in)  "<LscmbbBrkDecel_A_Rq>"
  bus_selector/8 -> LscmbbBrkDecel_B_Enbl/1(in)  "<LscmbbBrkDecel_B_Enbl>"
  bus_selector/9 -> LscmbbBrkDecel_No_Cnt/1(in)  "<LscmbbBrkDecel_No_Cnt>"
  bus_selector/10 -> LscmbbBrkDecel_No_Cs/1(in)  "<LscmbbBrkDecel_No_Cs>"
  bus_selector/11 -> LscmbbBrkPrchg_D_Rq/1(in)  "<LscmbbBrkPrchg_D_Rq>"
  bus_selector/12 -> LscmbbDeny_B_Actl/1(in)  "<LscmbbDeny_B_Actl>"
  bus_selector/13 -> LscmbbEngTqMn_B_Rq/1(in)  "<LscmbbEngTqMn_B_Rq>"
  bus_selector/14 -> LscmbbMsgTxt_D_Rq/1(in)  "<LscmbbMsgTxt_D_Rq>"
  bus_selector/15 -> LscmbbPostEvnt_B_Dsply/1(in)  "<LscmbbPostEvnt_B_Dsply>"
  bus_selector/16 -> LscmbbSrvcRqd_B_Rq/1(in)  "<LscmbbSrvcRqd_B_Rq>"
  bus_selector/17 -> WndwFrontHeat_B_Rq/1(in)  "<WndwFrontHeat_B_Rq>"
  in/1 -> bus_selector/1

== system test_mdl_NI/CAN_Signal/GWM/Other_GWMTx/GGCC_Config_Mgmt_ID_1_FD1 ==
  in : Inport
  VehicleGGCCData : Subsystem
  bus_creator : BusCreator  Inputs=1
  bus_selector : BusSelector  OutputSignals=VehicleGGCCData
  out_port : Outport
  wires:
  bus_creator/1 -> out_port/1  "GGCC_Config_Mgmt_ID_1_FD1"
  VehicleGGCCData/1(out) -> bus_creator/1  "VehicleGGCCData"
  bus_selector/1 -> VehicleGGCCData/1(in)  "<VehicleGGCCData>"
  in/1 -> bus_selector/1

== system test_mdl_NI/CAN_Signal/GWM/Other_GWMTx/GWM_AutoSar_NetMgmt_FD1 ==
  in : Inport
  GWM_AutoSarNMControl : Subsystem
  GWM_AutoSarNMNodeId : Subsystem
  GWM_AutoSarNMReserved1 : Subsystem
  GWM_AutoSarNMReserved2 : Subsystem
  GWM_AutoSarNMReserved3 : Subsystem
  GWM_AutoSarNMReserved4 : Subsystem
  GWM_GWNMProxy : Subsystem
  GWM_GWOnBoardTester : Subsystem
  bus_creator : BusCreator  Inputs=8
  bus_selector : BusSelector  OutputSignals=GWM_AutoSarNMControl,GWM_AutoSarNMNodeId,GWM_AutoSarNMReserved1,GWM_AutoSarNMReserved2,GWM_AutoSarNMReserved3,GWM_AutoSarNMReserved4,GWM_GWNMProxy,GWM_GWOnBoardTester
  out_port : Outport
  wires:
  bus_creator/1 -> out_port/1  "GWM_AutoSar_NetMgmt_FD1"
  GWM_AutoSarNMControl/1(out) -> bus_creator/1  "GWM_AutoSarNMControl"
  GWM_AutoSarNMNodeId/1(out) -> bus_creator/2  "GWM_AutoSarNMNodeId"
  GWM_AutoSarNMReserved1/1(out) -> bus_creator/3  "GWM_AutoSarNMReserved1"
  GWM_AutoSarNMReserved2/1(out) -> bus_creator/4  "GWM_AutoSarNMReserved2"
  GWM_AutoSarNMReserved3/1(out) -> bus_creator/5  "GWM_AutoSarNMReserved3"
  GWM_AutoSarNMReserved4/1(out) -> bus_creator/6  "GWM_AutoSarNMReserved4"
  GWM_GWNMProxy/1(out) -> bus_creator/7  "GWM_GWNMProxy"
  GWM_GWOnBoardTester/1(out) -> bus_creator/8  "GWM_GWOnBoardTester"
  bus_selector/1 -> GWM_AutoSarNMControl/1(in)  "<GWM_AutoSarNMControl>"
  bus_selector/2 -> GWM_AutoSarNMNodeId/1(in)  "<GWM_AutoSarNMNodeId>"
  bus_selector/3 -> GWM_AutoSarNMReserved1/1(in)  "<GWM_AutoSarNMReserved1>"
  bus_selector/4 -> GWM_AutoSarNMReserved2/1(in)  "<GWM_AutoSarNMReserved2>"
  bus_selector/5 -> GWM_AutoSarNMReserved3/1(in)  "<GWM_AutoSarNMReserved3>"
  bus_selector/6 -> GWM_AutoSarNMReserved4/1(in)  "<GWM_AutoSarNMReserved4>"
  bus_selector/7 -> GWM_GWNMProxy/1(in)  "<GWM_GWNMProxy>"
  bus_selector/8 -> GWM_GWOnBoardTester/1(in)  "<GWM_GWOnBoardTester>"
  in/1 -> bus_selector/1

== system test_mdl_NI/CAN_Signal/GWM/Other_GWMTx/GlobalClock_Data_FD1 ==
  in : Inport
  GlblClkDay_No_Actl : Subsystem
  GlblClkHr_No_Actl : Subsystem
  GlblClkMnte_No_Actl : Subsystem
  GlblClkScnd_No_Actl : Subsystem
  GlblClkYr_No_Actl : Subsystem
  bus_creator : BusCreator  Inputs=5
  bus_selector : BusSelector  OutputSignals=GlblClkDay_No_Actl,GlblClkHr_No_Actl,GlblClkMnte_No_Actl,GlblClkScnd_No_Actl,GlblClkYr_No_Actl
  out_port : Outport
  wires:
  bus_creator/1 -> out_port/1  "GlobalClock_Data_FD1"
  GlblClkDay_No_Actl/1(out) -> bus_creator/1  "GlblClkDay_No_Actl"
  GlblClkHr_No_Actl/1(out) -> bus_creator/2  "GlblClkHr_No_Actl"
  GlblClkMnte_No_Actl/1(out) -> bus_creator/3  "GlblClkMnte_No_Actl"
  GlblClkScnd_No_Actl/1(out) -> bus_creator/4  "GlblClkScnd_No_Actl"
  GlblClkYr_No_Actl/1(out) -> bus_creator/5  "GlblClkYr_No_Actl"
  bus_selector/1 -> GlblClkDay_No_Actl/1(in)  "<GlblClkDay_No_Actl>"
  bus_selector/2 -> GlblClkHr_No_Actl/1(in)  "<GlblClkHr_No_Actl>"
  bus_selector/3 -> GlblClkMnte_No_Actl/1(in)  "<GlblClkMnte_No_Actl>"
  bus_selector/4 -> GlblClkScnd_No_Actl/1(in)  "<GlblClkScnd_No_Actl>"
  bus_selector/5 -> GlblClkYr_No_Actl/1(in)  "<GlblClkYr_No_Actl>"
  in/1 -> bus_selector/1

== system test_mdl_NI/CAN_Signal/GWM/Other_GWMTx/Global_PATS_Cntrl_Info_FD1 ==
  in : Inport
  bus_creator : BusCreator  Inputs=2
  bus_selector : BusSelector  OutputSignals=immoControlCmd_T1,immoControlData_T1
  immoControlCmd_T1 : Subsystem
  immoControlData_T1 : Subsystem
  out_port : Outport
  wires:
  bus_creator/1 -> out_port/1  "Global_PATS_Cntrl_Info_FD1"
  immoControlCmd_T1/1(out) -> bus_creator/1  "immoControlCmd_T1"
  immoControlData_T1/1(out) -> bus_creator/2  "immoControlData_T1"
  bus_selector/1 -> immoControlCmd_T1/1(in)  "<immoControlCmd_T1>"
  bus_selector/2 -> immoControlData_T1/1(in)  "<immoControlData_T1>"
  in/1 -> bus_selector/1

== system test_mdl_NI/CAN_Signal/GWM/Other_GWMTx/IPC_Infotainment_FD1 ==
  in : Inport
  BeltminderAudioMute : Subsystem
  Chime_Source : Subsystem
  HdcOn_B_Rq : Subsystem
  IPC_Attn_Info_Audio : Subsystem
  IPC_MyKeyVolLimit_St : Subsystem
  IPC_New_Attn_Event : Subsystem
  Power_Up_Chime_Modules : Subsystem
  Veh_V2_Dsply : Subsystem
  bus_creator : BusCreator  Inputs=8
  bus_selector : BusSelector  OutputSignals=BeltminderAudioMute,Chime_Source,HdcOn_B_Rq,IPC_Attn_Info_Audio,IPC_MyKeyVolLimit_St,IPC_New_Attn_Event,Power_Up_Chime_Modules,Veh_V2_Dsply
  out_port : Outport
  wires:
  bus_creator/1 -> out_port/1  "IPC_Infotainment_FD1"
  BeltminderAudioMute/1(out) -> bus_creator/1  "BeltminderAudioMute"
  Chime_Source/1(out) -> bus_creator/2  "Chime_Source"
  HdcOn_B_Rq/1(out) -> bus_creator/3  "HdcOn_B_Rq"
  IPC_Attn_Info_Audio/1(out) -> bus_creator/4  "IPC_Attn_Info_Audio"
  IPC_MyKeyVolLimit_St/1(out) -> bus_creator/5  "IPC_MyKeyVolLimit_St"
  IPC_New_Attn_Event/1(out) -> bus_creator/6  "IPC_New_Attn_Event"
  Power_Up_Chime_Modules/1(out) -> bus_creator/7  "Power_Up_Chime_Modules"
  Veh_V2_Dsply/1(out) -> bus_creator/8  "Veh_V2_Dsply"
  bus_selector/1 -> BeltminderAudioMute/1(in)  "<BeltminderAudioMute>"
  bus_selector/2 -> Chime_Source/1(in)  "<Chime_Source>"
  bus_selector/3 -> HdcOn_B_Rq/1(in)  "<HdcOn_B_Rq>"
  bus_selector/4 -> IPC_Attn_Info_Audio/1(in)  "<IPC_Attn_Info_Audio>"
  bus_selector/5 -> IPC_MyKeyVolLimit_St/1(in)  "<IPC_MyKeyVolLimit_St>"
  bus_selector/6 -> IPC_New_Attn_Event/1(in)  "<IPC_New_Attn_Event>"
  bus_selector/7 -> Power_Up_Chime_Modules/1(in)  "<Power_Up_Chime_Modules>"
  bus_selector/8 -> Veh_V2_Dsply/1(in)  "<Veh_V2_Dsply>"
  in/1 -> bus_selector/1

== system test_mdl_NI/CAN_Signal/GWM/Other_GWMTx/IPC_Send_Signals_2_FD1 ==
  in : Inport
  ElLongTerm_L_Dsply : Subsystem
  ElTrip_L_Dsply : Subsystem
  FuelRange_L_Dsply : Subsystem
  bus_creator : BusCreator  Inputs=3
  bus_selector : BusSelector  OutputSignals=ElLongTerm_L_Dsply,ElTrip_L_Dsply,FuelRange_L_Dsply
  out_port : Outport
  wires:
  bus_creator/1 -> out_port/1  "IPC_Send_Signals_2_FD1"
  ElLongTerm_L_Dsply/1(out) -> bus_creator/1  "ElLongTerm_L_Dsply"
  ElTrip_L_Dsply/1(out) -> bus_creator/2  "ElTrip_L_Dsply"
  FuelRange_L_Dsply/1(out) -> bus_creator/3  "FuelRange_L_Dsply"
  bus_selector/1 -> ElLongTerm_L_Dsply/1(in)  "<ElLongTerm_L_Dsply>"
  bus_selector/2 -> ElTrip_L_Dsply/1(in)  "<ElTrip_L_Dsply>"
  bus_selector/3 -> FuelRange_L_Dsply/1(in)  "<FuelRange_L_Dsply>"
  in/1 -> bus_selector/1

== system test_mdl_NI/CAN_Signal/GWM/Other_GWMTx/MHT_EV_Wakeup_FD1 ==
  in : Inport
  BattChlrSov_B_Rq : Subsystem
  BattChrgTrgtSoC_D_Rq : Subsystem
  BattTracDrvSustn_B_Rq : Subsystem
  BrkAppl_D_RqPt : Subsystem
  CabnEvapSovFront_B_Rq : Subsystem
  CabnEvapSovRear_B_Rq : Subsystem
  HeatCoreSovRear_B_Rq : Subsystem
  HtrnClntFlw_D_Rq : Subsystem
  HtrnCnnctPwr_B_Stat : Subsystem
  HtrnDcdcDis_B_Rq : Subsystem
  PtcHtr_D_Stat : Subsystem
  bus_creator : BusCreator  Inputs=11
  bus_selector : BusSelector  OutputSignals=BattChlrSov_B_Rq,BattChrgTrgtSoC_D_Rq,BattTracDrvSustn_B_Rq,BrkAppl_D_RqPt,CabnEvapSovFront_B_Rq,CabnEvapSovRear_B_Rq,HeatCoreSovRear_B_Rq,HtrnClntFlw_D_Rq,HtrnCnnctPwr_B_Stat,HtrnDcdcDis_B_Rq,PtcHtr_D_Stat
  out_port : Outport
  wires:
  bus_creator/1 -> out_port/1  "MHT_EV_Wakeup_FD1"
  BattChlrSov_B_Rq/1(out) -> bus_creator/1  "BattChlrSov_B_Rq"
  BattChrgTrgtSoC_D_Rq/1(out) -> bus_creator/2  "BattChrgTrgtSoC_D_Rq"
  BattTracDrvSustn_B_Rq/1(out) -> bus_creator/3  "BattTracDrvSustn_B_Rq"
  BrkAppl_D_RqPt/1(out) -> bus_creator/4  "BrkAppl_D_RqPt"
  CabnEvapSovFront_B_Rq/1(out) -> bus_creator/5  "CabnEvapSovFront_B_Rq"
  CabnEvapSovRear_B_Rq/1(out) -> bus_creator/6  "CabnEvapSovRear_B_Rq"
  HeatCoreSovRear_B_Rq/1(out) -> bus_creator/7  "HeatCoreSovRear_B_Rq"
  HtrnClntFlw_D_Rq/1(out) -> bus_creator/8  "HtrnClntFlw_D_Rq"
  HtrnCnnctPwr_B_Stat/1(out) -> bus_creator/9  "HtrnCnnctPwr_B_Stat"
  HtrnDcdcDis_B_Rq/1(out) -> bus_creator/10  "HtrnDcdcDis_B_Rq"
  PtcHtr_D_Stat/1(out) -> bus_creator/11  "PtcHtr_D_Stat"
  bus_selector/1 -> BattChlrSov_B_Rq/1(in)  "<BattChlrSov_B_Rq>"
  bus_selector/2 -> BattChrgTrgtSoC_D_Rq/1(in)  "<BattChrgTrgtSoC_D_Rq>"
  bus_selector/3 -> BattTracDrvSustn_B_Rq/1(in)  "<BattTracDrvSustn_B_Rq>"
  bus_selector/4 -> BrkAppl_D_RqPt/1(in)  "<BrkAppl_D_RqPt>"
  bus_selector/5 -> CabnEvapSovFront_B_Rq/1(in)  "<CabnEvapSovFront_B_Rq>"
  bus_selector/6 -> CabnEvapSovRear_B_Rq/1(in)  "<CabnEvapSovRear_B_Rq>"
  bus_selector/7 -> HeatCoreSovRear_B_Rq/1(in)  "<HeatCoreSovRear_B_Rq>"
  bus_selector/8 -> HtrnClntFlw_D_Rq/1(in)  "<HtrnClntFlw_D_Rq>"
  bus_selector/9 -> HtrnCnnctPwr_B_Stat/1(in)  "<HtrnCnnctPwr_B_Stat>"
  bus_selector/10 -> HtrnDcdcDis_B_Rq/1(in)  "<HtrnDcdcDis_B_Rq>"
  bus_selector/11 -> PtcHtr_D_Stat/1(in)  "<PtcHtr_D_Stat>"
  in/1 -> bus_selector/1

== system test_mdl_NI/CAN_Signal/GWM/Other_GWMTx/Mc_Send_Signals_2_FD1 ==
  in : Inport
  BttOn_B_Rq : Subsystem
  Btt_L_Actl : Subsystem
  EngExhMdeQuiet_D_Rq : Subsystem
  EsaOn_B_Rq : Subsystem
  Mc_VehLangUsrSel_St : Subsystem
  Mc_VehUnitTempUsrSel_St : Subsystem
  Mc_VehUntTrpCoUsrSel_St : Subsystem
  SelDrvMdeDsply_B_Avail : Subsystem
  SelDrvMdeTxtReset_B_Rq : Subsystem
  WaitToStartLamp_D_Falt : Subsystem
  bus_creator : BusCreator  Inputs=10
  bus_selector : BusSelector  OutputSignals=BttOn_B_Rq,Btt_L_Actl,EngExhMdeQuiet_D_Rq,EsaOn_B_Rq,Mc_VehLangUsrSel_St,Mc_VehUnitTempUsrSel_St,Mc_VehUntTrpCoUsrSel_St,SelDrvMdeDsply_B_Avail,SelDrvMdeTxtReset_B_Rq,WaitToStartLamp_D_Falt
  out_port : Outport
  wires:
  bus_creator/1 -> out_port/1  "Mc_Send_Signals_2_FD1"
  BttOn_B_Rq/1(out) -> bus_creator/1  "BttOn_B_Rq"
  Btt_L_Actl/1(out) -> bus_creator/2  "Btt_L_Actl"
  EngExhMdeQuiet_D_Rq/1(out) -> bus_creator/3  "EngExhMdeQuiet_D_Rq"
  EsaOn_B_Rq/1(out) -> bus_creator/4  "EsaOn_B_Rq"
  Mc_VehLangUsrSel_St/1(out) -> bus_creator/5  "Mc_VehLangUsrSel_St"
  Mc_VehUnitTempUsrSel_St/1(out) -> bus_creator/6  "Mc_VehUnitTempUsrSel_St"
  Mc_VehUntTrpCoUsrSel_St/1(out) -> bus_creator/7  "Mc_VehUntTrpCoUsrSel_St"
  SelDrvMdeDsply_B_Avail/1(out) -> bus_creator/8  "SelDrvMdeDsply_B_Avail"
  SelDrvMdeTxtReset_B_Rq/1(out) -> bus_creator/9  "SelDrvMdeTxtReset_B_Rq"
  WaitToStartLamp_D_Falt/1(out) -> bus_creator/10  "WaitToStartLamp_D_Falt"
  bus_selector/1 -> BttOn_B_Rq/1(in)  "<BttOn_B_Rq>"
  bus_selector/2 -> Btt_L_Actl/1(in)  "<Btt_L_Actl>"
  bus_selector/3 -> EngExhMdeQuiet_D_Rq/1(in)  "<EngExhMdeQuiet_D_Rq>"
  bus_selector/4 -> EsaOn_B_Rq/1(in)  "<EsaOn_B_Rq>"
  bus_selector/5 -> Mc_VehLangUsrSel_St/1(in)  "<Mc_VehLangUsrSel_St>"
  bus_selector/6 -> Mc_VehUnitTempUsrSel_St/1(in)  "<Mc_VehUnitTempUsrSel_St>"
  bus_selector/7 -> Mc_VehUntTrpCoUsrSel_St/1(in)  "<Mc_VehUntTrpCoUsrSel_St>"
  bus_selector/8 -> SelDrvMdeDsply_B_Avail/1(in)  "<SelDrvMdeDsply_B_Avail>"
  bus_selector/9 -> SelDrvMdeTxtReset_B_Rq/1(in)  "<SelDrvMdeTxtReset_B_Rq>"
  bus_selector/10 -> WaitToStartLamp_D_Falt/1(in)  "<WaitToStartLamp_D_Falt>"
  in/1 -> bus_selector/1

== system test_mdl_NI/CAN_Signal/GWM/Other_GWMTx/ParkAid_Aud_Warn_CmdM_FD1 ==
  in : Inport
  Cta_D_Rq : Subsystem
  PrkAidRear_D_RqDrv : Subsystem
  Sod_D_Rq : Subsystem
  SteEffort_D_Rq : Subsystem
  bus_creator : BusCreator  Inputs=4
  bus_selector : BusSelector  OutputSignals=Cta_D_Rq,PrkAidRear_D_RqDrv,Sod_D_Rq,SteEffort_D_Rq
  out_port : Outport
  wires:
  bus_creator/1 -> out_port/1  "ParkAid_Aud_Warn_CmdM_FD1"
  Cta_D_Rq/1(out) -> bus_creator/1  "Cta_D_Rq"
  PrkAidRear_D_RqDrv/1(out) -> bus_creator/2  "PrkAidRear_D_RqDrv"
  Sod_D_Rq/1(out) -> bus_creator/3  "Sod_D_Rq"
  SteEffort_D_Rq/1(out) -> bus_creator/4  "SteEffort_D_Rq"
  bus_selector/1 -> Cta_D_Rq/1(in)  "<Cta_D_Rq>"
  bus_selector/2 -> PrkAidRear_D_RqDrv/1(in)  "<PrkAidRear_D_RqDrv>"
  bus_selector/3 -> Sod_D_Rq/1(in)  "<Sod_D_Rq>"
  bus_selector/4 -> SteEffort_D_Rq/1(in)  "<SteEffort_D_Rq>"
  in/1 -> bus_selector/1

== system test_mdl_NI/CAN_Signal/GWM/Other_GWMTx/Pass_Dr_Stat_FD1 ==
  in : Inport
  BLISLEDStatPassSide : Subsystem
  ChildLckFdbckRp_B_Stat : Subsystem
  Memory_1_SwPsngr_Stat : Subsystem
  Memory_2_SwPsngr_Stat : Subsystem
  Memory_3_SwPsngr_Stat : Subsystem
  Pasngr_Lock_Sw_Cnt : Subsystem
  Pasngr_Lock_Sw_Stat : Subsystem
  RollCode_No_ActlPdm : Subsystem
  WndwPsngrSide_D_Stat : Subsystem
  bus_creator : BusCreator  Inputs=9
  bus_selector : BusSelector  OutputSignals=BLISLEDStatPassSide,ChildLckFdbckRp_B_Stat,Memory_1_SwPsngr_Stat,Memory_2_SwPsngr_Stat,Memory_3_SwPsngr_Stat,Pasngr_Lock_Sw_Cnt,Pasngr_Lock_Sw_Stat,RollCode_No_ActlPdm,WndwPsngrSide_D_Stat
  out_port : Outport
  wires:
  bus_creator/1 -> out_port/1  "Pass_Dr_Stat_FD1"
  BLISLEDStatPassSide/1(out) -> bus_creator/1  "BLISLEDStatPassSide"
  ChildLckFdbckRp_B_Stat/1(out) -> bus_creator/2  "ChildLckFdbckRp_B_Stat"
  Memory_1_SwPsngr_Stat/1(out) -> bus_creator/3  "Memory_1_SwPsngr_Stat"
  Memory_2_SwPsngr_Stat/1(out) -> bus_creator/4  "Memory_2_SwPsngr_Stat"
  Memory_3_SwPsngr_Stat/1(out) -> bus_creator/5  "Memory_3_SwPsngr_Stat"
  Pasngr_Lock_Sw_Cnt/1(out) -> bus_creator/6  "Pasngr_Lock_Sw_Cnt"
  Pasngr_Lock_Sw_Stat/1(out) -> bus_creator/7  "Pasngr_Lock_Sw_Stat"
  RollCode_No_ActlPdm/1(out) -> bus_creator/8  "RollCode_No_ActlPdm"
  WndwPsngrSide_D_Stat/1(out) -> bus_creator/9  "WndwPsngrSide_D_Stat"
  bus_selector/1 -> BLISLEDStatPassSide/1(in)  "<BLISLEDStatPassSide>"
  bus_selector/2 -> ChildLckFdbckRp_B_Stat/1(in)  "<ChildLckFdbckRp_B_Stat>"
  bus_selector/3 -> Memory_1_SwPsngr_Stat/1(in)  "<Memory_1_SwPsngr_Stat>"
  bus_selector/4 -> Memory_2_SwPsngr_Stat/1(in)  "<Memory_2_SwPsngr_Stat>"
  bus_selector/5 -> Memory_3_SwPsngr_Stat/1(in)  "<Memory_3_SwPsngr_Stat>"
  bus_selector/6 -> Pasngr_Lock_Sw_Cnt/1(in)  "<Pasngr_Lock_Sw_Cnt>"
  bus_selector/7 -> Pasngr_Lock_Sw_Stat/1(in)  "<Pasngr_Lock_Sw_Stat>"
  bus_selector/8 -> RollCode_No_ActlPdm/1(in)  "<RollCode_No_ActlPdm>"
  bus_selector/9 -> WndwPsngrSide_D_Stat/1(in)  "<WndwPsngrSide_D_Stat>"
  in/1 -> bus_selector/1

== system test_mdl_NI/CAN_Signal/GWM/Other_GWMTx/Personality_APIM_Data_FD1 ==
  in : Inport
  CtrStkDsplyOp_D_Rq : Subsystem
  CtrStkFeatConfigActl : Subsystem
  CtrStkFeatNoActl : Subsystem
  CtrStkPersIndex_D_Actl : Subsystem
  Pers1OptIn_B_Stats : Subsystem
  Pers2OptIn_B_Stats : Subsystem
  Pers3OptIn_B_Stats : Subsystem
  Pers4OptIn_B_Stats : Subsystem
  PersStore_D_Rq : Subsystem
  bus_creator : BusCreator  Inputs=9
  bus_selector : BusSelector  OutputSignals=CtrStkDsplyOp_D_Rq,CtrStkFeatConfigActl,CtrStkFeatNoActl,CtrStkPersIndex_D_Actl,Pers1OptIn_B_Stats,Pers2OptIn_B_Stats,Pers3OptIn_B_Stats,Pers4OptIn_B_Stats,PersStore_D_Rq
  out_port : Outport
  wires:
  bus_creator/1 -> out_port/1  "Personality_APIM_Data_FD1"
  CtrStkDsplyOp_D_Rq/1(out) -> bus_creator/1  "CtrStkDsplyOp_D_Rq"
  CtrStkFeatConfigActl/1(out) -> bus_creator/2  "CtrStkFeatConfigActl"
  CtrStkFeatNoActl/1(out) -> bus_creator/3  "CtrStkFeatNoActl"
  CtrStkPersIndex_D_Actl/1(out) -> bus_creator/4  "CtrStkPersIndex_D_Actl"
  Pers1OptIn_B_Stats/1(out) -> bus_creator/5  "Pers1OptIn_B_Stats"
  Pers2OptIn_B_Stats/1(out) -> bus_creator/6  "Pers2OptIn_B_Stats"
  Pers3OptIn_B_Stats/1(out) -> bus_creator/7  "Pers3OptIn_B_Stats"
  Pers4OptIn_B_Stats/1(out) -> bus_creator/8  "Pers4OptIn_B_Stats"
  PersStore_D_Rq/1(out) -> bus_creator/9  "PersStore_D_Rq"
  bus_selector/1 -> CtrStkDsplyOp_D_Rq/1(in)  "<CtrStkDsplyOp_D_Rq>"
  bus_selector/2 -> CtrStkFeatConfigActl/1(in)  "<CtrStkFeatConfigActl>"
  bus_selector/3 -> CtrStkFeatNoActl/1(in)  "<CtrStkFeatNoActl>"
  bus_selector/4 -> CtrStkPersIndex_D_Actl/1(in)  "<CtrStkPersIndex_D_Actl>"
  bus_selector/5 -> Pers1OptIn_B_Stats/1(in)  "<Pers1OptIn_B_Stats>"
  bus_selector/6 -> Pers2OptIn_B_Stats/1(in)  "<Pers2OptIn_B_Stats>"
  bus_selector/7 -> Pers3OptIn_B_Stats/1(in)  "<Pers3OptIn_B_Stats>"
  bus_selector/8 -> Pers4OptIn_B_Stats/1(in)  "<Pers4OptIn_B_Stats>"
  bus_selector/9 -> PersStore_D_Rq/1(in)  "<PersStore_D_Rq>"
  in/1 -> bus_selector/1

== system test_mdl_NI/CAN_Signal/GWM/Other_GWMTx/Personality_Data_FD1 ==
  in : Inport
  MsgCntrDsplyOp_D_Rq : Subsystem
  MsgCntrFeatConfigRq : Subsystem
  MsgCntrFeatNoRq : Subsystem
  MsgCntrPersIndex_D_Rq : Subsystem
  bus_creator : BusCreator  Inputs=4
  bus_selector : BusSelector  OutputSignals=MsgCntrDsplyOp_D_Rq,MsgCntrFeatConfigRq,MsgCntrFeatNoRq,MsgCntrPersIndex_D_Rq
  out_port : Outport
  wires:
  bus_creator/1 -> out_port/1  "Personality_Data_FD1"
  MsgCntrDsplyOp_D_Rq/1(out) -> bus_creator/1  "MsgCntrDsplyOp_D_Rq"
  MsgCntrFeatConfigRq/1(out) -> bus_creator/2  "MsgCntrFeatConfigRq"
  MsgCntrFeatNoRq/1(out) -> bus_creator/3  "MsgCntrFeatNoRq"
  MsgCntrPersIndex_D_Rq/1(out) -> bus_creator/4  "MsgCntrPersIndex_D_Rq"
  bus_selector/1 -> MsgCntrDsplyOp_D_Rq/1(in)  "<MsgCntrDsplyOp_D_Rq>"
  bus_selector/2 -> MsgCntrFeatConfigRq/1(in)  "<MsgCntrFeatConfigRq>"
  bus_selector/3 -> MsgCntrFeatNoRq/1(in)  "<MsgCntrFeatNoRq>"
  bus_selector/4 -> MsgCntrPersIndex_D_Rq/1(in)  "<MsgCntrPersIndex_D_Rq>"
  in/1 -> bus_selector/1

== system test_mdl_NI/CAN_Signal/GWM/Other_GWMTx/Power_Liftgate_Stat_FD1 ==
  in : Inport
  DrLckCnt_No_ActlTgate : Subsystem
  DrTGate_D_Rq : Subsystem
  DrTgateChime2_D_Rq : Subsystem
  Power_Liftgate_Mode_Stt : Subsystem
  PwLftgtIntSw_B_Stat : Subsystem
  bus_creator : BusCreator  Inputs=5
  bus_selector : BusSelector  OutputSignals=DrLckCnt_No_ActlTgate,DrTGate_D_Rq,DrTgateChime2_D_Rq,Power_Liftgate_Mode_Stt,PwLftgtIntSw_B_Stat
  out_port : Outport
  wires:
  bus_creator/1 -> out_port/1  "Power_Liftgate_Stat_FD1"
  DrLckCnt_No_ActlTgate/1(out) -> bus_creator/1  "DrLckCnt_No_ActlTgate"
  DrTGate_D_Rq/1(out) -> bus_creator/2  "DrTGate_D_Rq"
  DrTgateChime2_D_Rq/1(out) -> bus_creator/3  "DrTgateChime2_D_Rq"
  Power_Liftgate_Mode_Stt/1(out) -> bus_creator/4  "Power_Liftgate_Mode_Stt"
  PwLftgtIntSw_B_Stat/1(out) -> bus_creator/5  "PwLftgtIntSw_B_Stat"
  bus_selector/1 -> DrLckCnt_No_ActlTgate/1(in)  "<DrLckCnt_No_ActlTgate>"
  bus_selector/2 -> DrTGate_D_Rq/1(in)  "<DrTGate_D_Rq>"
  bus_selector/3 -> DrTgateChime2_D_Rq/1(in)  "<DrTgateChime2_D_Rq>"
  bus_selector/4 -> Power_Liftgate_Mode_Stt/1(in)  "<Power_Liftgate_Mode_Stt>"
  bus_selector/5 -> PwLftgtIntSw_B_Stat/1(in)  "<PwLftgtIntSw_B_Stat>"
  in/1 -> bus_selector/1

== system test_mdl_NI/CAN_Signal/GWM/Other_GWMTx/PreCond_Hev_Data1_FD1 ==
  in : Inport
  ChrgStat_D2_Dsply : Subsystem
  bus_creator : BusCreator  Inputs=1
  bus_selector : BusSelector  OutputSignals=ChrgStat_D2_Dsply
  out_port : Outport
  wires:
  bus_creator/1 -> out_port/1  "PreCond_Hev_Data1_FD1"
  ChrgStat_D2_Dsply/1(out) -> bus_creator/1  "ChrgStat_D2_Dsply"
  bus_selector/1 -> ChrgStat_D2_Dsply/1(in)  "<ChrgStat_D2_Dsply>"
  in/1 -> bus_selector/1
